simulink model "final_lane_following_model"  (R2024a)
settings: Solver=VariableStepAuto  StartTime=0.0  StopTime=5  RelTol=1e-3
model workspace (MAT data in the model file):
  polmodel = idpoly
  polmodel.IOSize_ = [0 0]
  polmodel.Data_ = idpack.polydata
  polmodel.Data_.Structure = pmodel.polynomial
  polmodel.Data_.Report = idresults.polyest
  polmodel.Data_.Report.Fit.FitPercent = []
  polmodel.Data_.Report.Fit.LossFcn = []
  polmodel.Data_.Report.Fit.MSE = []
  polmodel.Data_.Report.Fit.FPE = []
  polmodel.Data_.Report.Fit.AIC = []
  polmodel.Data_.Report.Fit.AICc = []
  polmodel.Data_.Report.Fit.nAIC = []
  polmodel.Data_.Report.Fit.BIC = []
  polmodel.Data_.Report.Parameters.ParVector = []
  polmodel.Data_.Report.Parameters.Free = []
  polmodel.Data_.Report.Parameters.Labels = {}
  polmodel.Data_.Report.Parameters.FreeParCovariance = []
  polmodel.Data_.Report.Parameters.InitialCondition = 'zero'
  polmodel.Data_.Report.DataUsed.Name = ''
  polmodel.Data_.Report.DataUsed.Type = ''
  polmodel.Data_.Report.DataUsed.Length = []
  polmodel.Data_.Report.DataUsed.Ts = []
  polmodel.Data_.Report.DataUsed.InterSample = ''
  polmodel.Data_.Report.DataUsed.InputOffset = []
  polmodel.Data_.Report.DataUsed.OutputOffset = []
  polmodel.Data_.EstimationStatus = -Inf
  polmodel.Data_.Delay.Input = []
  polmodel.Data_.Delay.Output = []
  polmodel.Data_.Ts = -1
undefined symbols (not defined in the file): DiscIntNeverNeededParam
libraries: simulink x1
settings Model: Creator=khushl  LastModifiedBy=khushl

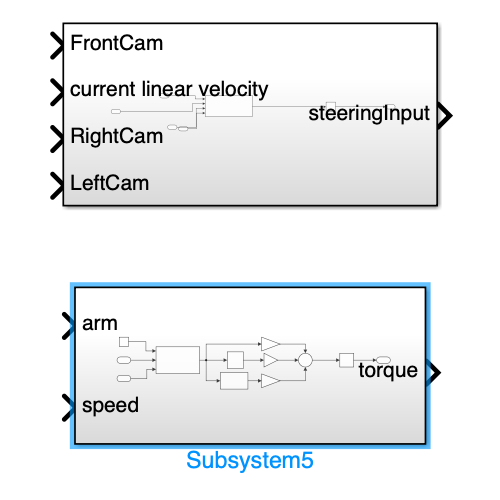
[thumbnail: Simulink's stored preview of the top-level diagram]
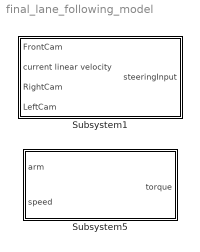
== system final_lane_following_model ==
  Subsystem1 : Subsystem
  Subsystem5 : Subsystem

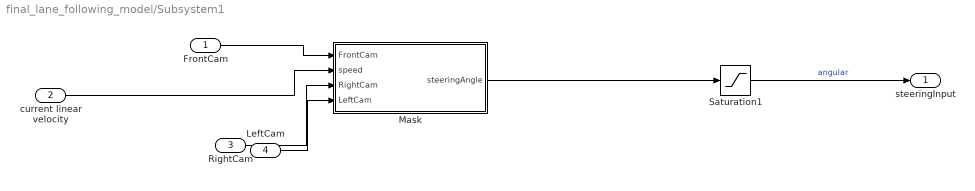
== system final_lane_following_model/Subsystem1 ==
  FrontCam : Inport
  current linear velocity : Inport  Port=2
  RightCam : Inport  Port=3
  LeftCam : Inport  Port=4
  Mask : MATLAB Function  TreatAsAtomicUnit=on
  Saturation1 : Saturate  UpperLimit=1  LowerLimit=-1
  steeringInput : Outport
  wires:
  current linear velocity/1 -> Mask/2(speed)
  Saturation1/1 -> steeringInput/1  "angular"
  FrontCam/1 -> Mask/1(FrontCam)
  Mask/1(steeringAngle) -> Saturation1/1
  RightCam/1 -> Mask/3(RightCam)
  LeftCam/1 -> Mask/4(LeftCam)

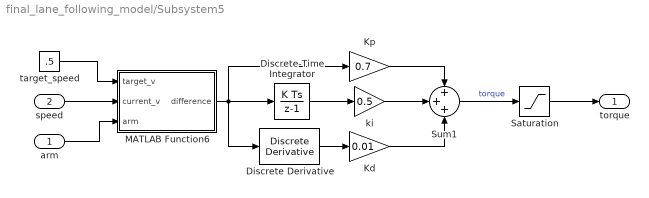
== system final_lane_following_model/Subsystem5 ==
  arm : Inport
  speed : Inport  Port=2
  Discrete Derivative : simulink/Discrete/Discrete Derivative  gainval=1.0  ICPrevScaledInput=0.0  OutMin=[]  OutMax=[2]  OutDataType=fixdt(1, 16)  OutScaling=2^-10  DoSatur=off
  Discrete-Time Integrator : DiscreteIntegrator  SampleTime=-1  LimitOutput=on  UpperSaturationLimit=2  LowerSaturationLimit=0  ICPrevOutput=DiscIntNeverNeededParam  ICPrevScaledInput=DiscIntNeverNeededParam
  Kd : Gain  Gain=0.01
  Kp : Gain  Gain=0.7
  MATLAB Function6 : MATLAB Function  TreatAsAtomicUnit=on
  Saturation : Saturate  UpperLimit=1  LowerLimit=0
  Sum1 : Sum  Inputs=+++
  ki : Gain  Gain=0.5
  target_speed : Constant  Value=.5  SampleTime=.1
  torque : Outport
  wires:
  target_speed/1 -> MATLAB Function6/1(target_v)
  arm/1 -> MATLAB Function6/3(arm)
  Sum1/1 -> Saturation/1  "torque"
  Discrete-Time Integrator/1 -> ki/1
  ki/1 -> Sum1/2
  Kp/1 -> Sum1/1
  Kd/1 -> Sum1/3
  MATLAB Function6/1(difference) -> Discrete-Time Integrator/1, Discrete Derivative/1, Kp/1
  Discrete Derivative/1 -> Kd/1
  Saturation/1 -> torque/1
  speed/1 -> MATLAB Function6/2(current_v)

== matlab function final_lane_following_model/Subsystem5/MATLAB Function6 ==
  data: target_v input; current_v input; arm input; difference output
function difference = fcn(target_v, current_v, arm)
    if arm == 1
       difference = target_v - current_v;
    else
       difference = 0;
    end
end

== matlab function final_lane_following_model/Subsystem1/Mask ==
  data: FrontCam input; steeringAngle output; speed input; RightCam input; LeftCam input
function steeringAngle  = processImage(FrontCam, speed, RightCam, LeftCam)
     % FrontCam = FrontCam*255;
     % RightCam=RightCam*255;
     % LeftCam=LeftCam*255;

    % Check for valid camera and speed inputs
    if FrontCam(1, 1, 1) == 0 && FrontCam(1, 1, 2) == 0 && FrontCam(1, 1, 3) == 0 || LeftCam(1, 1, 1) == 0 && LeftCam(1, 1, 2) == 0 && LeftCam(1, 1, 3) == 0 || RightCam(1, 1, 1) == 0 && RightCam(1, 1, 2) == 0 && RightCam(1, 1, 3) == 0
        steeringAngle = 0;
        return;
    end
    if speed == 0
        steeringAngle = 0;
        return;
    end

    % Downsampling the image inputs
    FrontCam = FrontCam(1:10:480, 1:10:640, :);
    LeftCam = LeftCam(1:10:480, 1:10:640, :);
    RightCam = RightCam(1:10:480, 1:10:640, :);

    % Define Camera Parameters
    height = 85;
    yaw = 0;
    pitch = 0;
    roll = 0;
    monoCams = cell(3, 1);
    
    % Camera intrinsics for resized images
    monoCams{1} = monoCamera(cameraIntrinsics([74.436956267387340,73.961386855604320],[32.280149907106400,25.661409210179094],[48,64]), height, ...
                                 "Pitch", pitch, ...
                                 "Yaw"  , yaw, ...
                                 "Roll" , roll, ...
                                 "SensorLocation", [0, 0],"WorldUnits", "millimeters");
    
    % monoCams{2} = monoCamera(cameraIntrinsics([1.195824753087169e+02,1.192432645881274e+02],[33.316484537512970,24.898802822108806],[48,64]), height, ...
    %                               "Pitch", pitch, ...
    %                               "Yaw"  , yaw, ...
    %                               "Roll" , roll, ...
    %                               "SensorLocation", [0, 0],"WorldUnits", "millimeters");
    % 
    % monoCams{3} = monoCamera(cameraIntrinsics([1.195824753087169e+02,1.192432645881274e+02],[33.316484537512970,24.898802822108806],[48,64]), height, ...
    %                               "Pitch", pitch, ...
    %                               "Yaw"  , yaw, ...
    %                               "Roll" , roll, ...
    %                               "SensorLocation", [0, 0],"WorldUnits", "millimeters");

    % Birds-Eye Transformation
    frontBevImgs  = transformImage(birdsEyeView(monoCams{1}, [200, 700, -250, 250], [64, NaN]), undistortImage(FrontCam, monoCams{1}.Intrinsics));

    FrontCam = frontBevImgs;
    
    

    % Color Thresholding for binary conversion
    channel1Min = 80.000;
    channel1Max = 255.000;
    channel2Min = 80.000;
    channel2Max = 255.000;
    channel3Min = 80.000;
    channel3Max = 255.000;
    
    % Convert FrontCam to binary image
    sliderBWFront = (FrontCam(:,:,1) >= channel1Min ) & (FrontCam(:,:,1) <= channel1Max) & ...
               (FrontCam(:,:,2) >= channel2Min ) & (FrontCam(:,:,2) <= channel2Max) & ...
               (FrontCam(:,:,3) >= channel3Min ) & (FrontCam(:,:,3) <= channel3Max);
    BWFront = sliderBWFront;
    BWFront = BWFront(end:-1:1, :);  % Flip the image vertically

    
    % Convert LeftCam to binary image
    sliderBWLeft = (LeftCam(:,:,1) >= channel1Min ) & (LeftCam(:,:,1) <= channel1Max) & ...
               (LeftCam(:,:,2) >= channel2Min ) & (LeftCam(:,:,2) <= channel2Max) & ...
               (LeftCam(:,:,3) >= channel3Min ) & (LeftCam(:,:,3) <= channel3Max);
    BWLeft = sliderBWLeft;
    BWLeft = BWLeft(end:-1:1, :);  % Flip the image vertically
    
    
    % Convert RightCam to binary image
    sliderBWRight = (RightCam(:,:,1) >= channel1Min ) & (RightCam(:,:,1) <= channel1Max) & ...
               (RightCam(:,:,2) >= channel2Min ) & (RightCam(:,:,2) <= channel2Max) & ...
               (RightCam(:,:,3) >= channel3Min ) & (RightCam(:,:,3) <= channel3Max);
    BWRight = sliderBWRight;
    BWRight = BWRight(end:-1:1, :);  % Flip the image vertically
    

    % Binning the binary images
    binnedFront = zeros(32, 32);
    
    for frontbinidx = 1:2:64
        for frontbinYidx = 1:2:64
            binnedFront(round(frontbinidx/2 + 0.5), round(frontbinYidx/2 + 0.5)) = max(BWFront(frontbinidx:frontbinidx+1, frontbinYidx:frontbinYidx+1), [], "all");
        end
    end
    
    binnedLeft = zeros(24, 32);
    
    for leftbinidx = 1:2:48
        for leftbinYidx = 1:2:64
            binnedLeft(round(leftbinidx/2 + 0.5), round(leftbinYidx/2 + 0.5)) = max(BWLeft(leftbinidx:leftbinidx+1, leftbinYidx:leftbinYidx+1), [], "all");
        end
    end
    
    binnedRight = zeros(24, 32);
    
    for rightbinidx = 1:2:48
        for rightbinYidx = 1:2:64
            binnedRight(round(rightbinidx/2 + 0.5), round(rightbinYidx/2 + 0.5)) = max(BWRight(rightbinidx:rightbinidx+1, rightbinYidx:rightbinYidx+1), [], "all");
        end
    end


    % Convert all coordinates from pixels to millimeters
    mm_per_pixel = 2.08;

    % Extract non-zero pixel coordinates for clustering
    [rows, cols] = find(binnedRight);
    RightCoordinates = [cols, rows] * mm_per_pixel;
    
    [rows, cols] = find(binnedLeft);
    LeftCoordinates = [cols, rows] * mm_per_pixel;
    
    offset_right = calculateOffsetFromCoordinates(RightCoordinates, 10);
    offset_left = calculateOffsetFromCoordinates(LeftCoordinates, 10)*-1;
    

    % Front Camera DBCAN and Transformation
    [rows, cols] = find(binnedFront);
    FrontCoordinates = [cols, rows];
    epsilon = 2;
    minPts = 3;
    minClusterSize = 10;
    maxClusterSize = 80;
    FrontClusters = dbscan(FrontCoordinates, epsilon, minPts);
    FrontUniqueClusters = unique(FrontClusters);
    FrontClusterSizes = histcounts(FrontClusters, [FrontUniqueClusters; max(FrontUniqueClusters)+1]);
    FrontmaxYRange = 0;
    FrontBestClusterIdx = -1;
    for iFront = 1:length(FrontUniqueClusters)
        FrontClusterIdx = (FrontClusters == FrontUniqueClusters(iFront));
        % Finding cluster within parameters with largest y-range
        if FrontClusterSizes(iFront) >= minClusterSize && FrontClusterSizes(iFront)<=maxClusterSize
            FrontClusterCoords = FrontCoordinates(FrontClusterIdx, :);
            FrontYRange = max(FrontClusterCoords(:, 2)) - min(FrontClusterCoords(:, 2));
            if FrontYRange > FrontmaxYRange
                FrontmaxYRange = FrontYRange;
                FrontBestClusterIdx = double(FrontUniqueClusters(iFront));
            end
        end
    end

    % Transforming coordinates to a x-axis birds eye view
    if FrontBestClusterIdx ~= -1
        FrontClusterIdx = (FrontClusters == FrontBestClusterIdx);
        FrontbestClusterCoords = FrontCoordinates(FrontClusterIdx, :);
        FrontTheta = 90;
        FrontR = [cosd(FrontTheta) -sind(FrontTheta); sind(FrontTheta) cosd(FrontTheta)];
        newFrontCoords = FrontbestClusterCoords * FrontR;
        newFrontCoords(:, 2) = newFrontCoords(:, 2) + 16;
        purePurs = polyfit(newFrontCoords(:,1), newFrontCoords(:,2), 3);
    else
        steeringAngle=0;
        return;
    end
    

    % Transformations for proper birds eye view
    % Front Camera: Move 215 mm forward
    % newFrontCoords(:, 1) = newFrontCoords(:, 1) + 215;
    % 
    % leftResult(:, 2) = leftResult(:, 2) + 173+75;
    % leftResult(:, 1) = leftResult(:, 1) + 30;
    % 
    % rightResult(:, 2) = rightResult(:, 2) *-1;
    % rightResult(:, 2) = rightResult(:, 2) -75-173;
    % rightResult(:, 1) = rightResult(:, 1) + 30;


    % Calculate steering angle using Pure Pursuit
    currentPos = [0, 0];
    lookahead_distance = 20;
    dx=lookahead_distance-currentPos(1);
    dy=polyval(purePurs, lookahead_distance)-currentPos(2);
    Lfw = sqrt(dx^2 + dy^2);
    mu = atan(dy / dx);
    if mu == 0
        steeringAngle = 0;
        return;
    end
    R = Lfw / (2 * sin(mu));
    arcLength = 2 * mu * R;
    time = arcLength / speed;
    steeringAngle = (2 * mu) / time;

    % Adding gain for steeringAngle and left/right offset
    gain = 51.5;
    offset_gain = 0.5;
    side_offset = (offset_right + offset_left)*offset_gain;
    steeringAngle = side_offset + steeringAngle * gain;
end

function offset = calculateOffsetFromCoordinates(coordinates, threshold)
    % Function to calculate offset based on the lowest y-value
    offset = 0;
    sortedCoords = sortrows(coordinates, 1);
    uniqueX = unique(sortedCoords(:, 1));
    result = zeros(length(uniqueX), 2);
    for i = 1:length(uniqueX)
        currentXIdx = (sortedCoords(:, 1) == uniqueX(i));
        minY = min(sortedCoords(currentXIdx, 2));
        result(i, :) = [uniqueX(i), minY];
    end
    lowestY = min(result(:, 2));
    if lowestY < threshold && lowestY > 0
        offset = 1 / lowestY;
    end
end
